simulink model "StepperMotorPullIn"  (R2023b)
settings: Solver=ode23t  StartTime=0.0  StopTime=timeSimulation  FixedStep=0.001  MaxStep=1/(4*numMicroStep*f*4)  RelTol=1e-3  AbsTol=1e-3  EnableMultiTasking=on
PreLoadFcn:
  | % Parameterize the stepper motor;
  | StepperMotorPullInData;
values from neighbouring files (symbols this model uses):
  CF = sqrt(2)    [StepperMotorPullInData.m]
  driveRampRate = -1/log(1-(1-exp(-1))/voltageFactor)    [StepperMotorPullInData.m]
  f = stepRate/4    (= 75)    [StepperMotorPullInData.m]    (also in StepperMotorPullInUpdatePlot.m = stepRateVector(i)/4)
  fullStepSize = 1.8    [StepperMotorPullInData.m]    (also in StepperMotorPullin.mat)
  inductance = 4.6    [StepperMotorPullInData.m]
  LF = 1    [StepperMotorPullInData.m]
  loadDamping = 0    [StepperMotorPullInData.m]
  loadTorque = 125    [StepperMotorPullInData.m]    (also in StepperMotorPullInUpdatePlot.m = (loadTorqueHigh+loadTorqueLow)/2)
  numMicroStep = 24    [StepperMotorPullInData.m]
  ratedCurrent = 1.2    [StepperMotorPullInData.m]
  resistance = 2.2    [StepperMotorPullInData.m]
  rotorDamping = 0.1e-3    (= 0.0001)    [StepperMotorPullInData.m]
  rotorInertia = 37e-7    (= 3.7e-06)    [StepperMotorPullInData.m]
  tolerance = 2    [StepperMotorPullInData.m]
libraries: fl_lib x16, nesl_utility x7, simulink x1, ee_lib x1
CloseFcn:
  | try,close(figHandleMotorStepper),end
  | clear figHandleMotorStepper
  | 
  | try,close(figHandlePlotMotorStepper),end
  | clear figHandlePlotMotorStepper;
  | 
  | clear simlog_StepperMotorPullin;
  | 
  | clear modelFileName ratedCurrent ratedVoltage resistance;
  | clear inductance fullStepSize holdingTorque detentTorque;
  | clear rotorInertia kTVal rotorDamping initialSpeed;
  | clear initialAngle numMicroStep driveVoltage voltageFactor;
  | clear driveRampRate CF loadDamping loadInertia;
  | clear LF numRotation tolerance torqueTolerance stepRateVector f;
  | clear plotXAxis stepRate loadTorque loadCycle numStep timeSimulation;
  | clear i nF torque stepRateVectorSimulated slipped;
  | clear loadTorqueLow loadTorqueHigh notFinished loadTorque;
  | clear torqueSingle stepRateVectorSingle figAxes;
  | clear strucAutoSaveOptions loadTorqueLowInitial loadTorqueHighInitial;
  | clear torqueDatasheet stepRateVectorDatasheet;
  | clear torqueSingle stepRateVectorSingle;
Description:
  | Stepper Motor Pull-in Characteristics
  | %
settings Model: Creator=The MathWorks, Inc.  LastModifiedBy=The MathWorks, Inc.
settings SolverCC: AlgebraicLoopSolver=TrustRegion
settings DataIOCC: MaxDataPoints=10000  SaveFormat=Array  SaveOutput=off  SignalLogging=off  DSMLogging=off  SaveTime=off  ReturnWorkspaceOutputs=off  SignalLoggingName=logsout_StepperMotor
settings OptimizationCC: ReuseModelBlockBuffer=off  ExpressionDepthLimit=2147483647  InitFltsAndDblsToZero=on  LifeSpan=inf
settings DebuggingCC: UnderspecifiedInitializationDetection=Classic  MergeDetectMultiDrivingBlocksExec=none  FcnCallInpInsideContextMsg=warning  UnconnectedInputMsg=warning  UnconnectedOutputMsg=warning  UnconnectedLineMsg=warning  StateNameClashWarn=warning  PregeneratedLibrarySubsystemCodeDiagnostic=none  SFUnexpectedBacktrackingDiag=warning  SFNoUnconditionalDefaultTransitionDiag=warning  SFExecutionAtInitializationDiag=none  ArithmeticOperatorsInVariantConditions=warning
settings HardwareCC: ProdBitPerPointer=32  ProdBitPerSizeT=32  ProdBitPerPtrDiffT=32  ProdLargestAtomicFloat=None  ProdIntDivRoundTo=Undefined  ProdEndianess=Unspecified  ProdWordSize=32  ProdHWDeviceType=32-bit Generic
settings ModelReferenceCC: EnableRefExpFcnMdlSchedulingChecks=on  PropagateSignalLabelsOutOfModel=off
settings SFSimCC: SimUseLocalCustomCode=off  CustomCodeUndefinedFunction=UseInterfaceOnly
settings RTWCC: RTWUseLocalCustomCode=off  DLArmComputeVersion=19.05
settings CodeAppCC: StateflowObjectComments=on
settings GRTTargetCC: TargetLangStandard=C89/C90 (ANSI)  CombineOutputUpdateFcns=off  GRTInterface=on
settings ConfigComp: CovScope=ReferencedModels  CovMetricSettings=dw  CovSaveCumulativeToWorkspaceVar=on  CovSaveSingleToWorkspaceVar=on  CovExternalEMLEnable=off  CovSFcnEnable=off
settings SimscapeCC: SimscapeLogType=all  SimscapeLogName=simlog_StepperMotorPullin  SimscapeLogLimitData=off

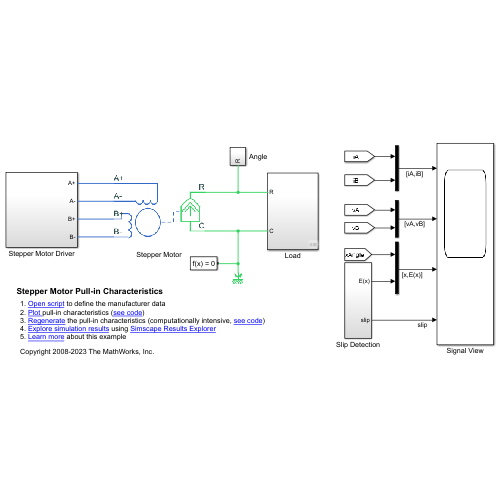
[thumbnail: Simulink's stored preview of the top-level diagram]
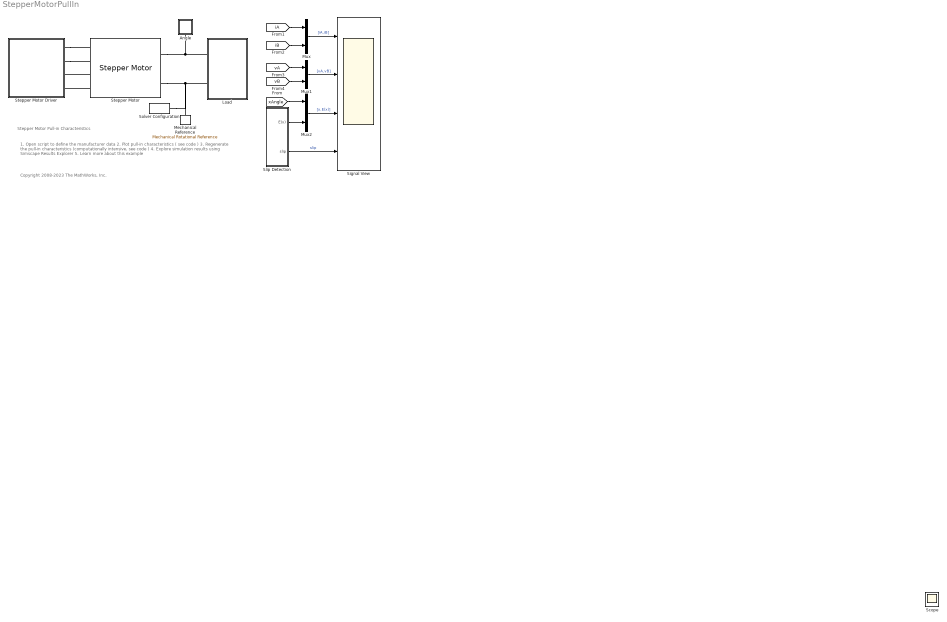
== system StepperMotorPullIn ==
  note: 1. Open script to define the manufacturer data
      | 2. Plot pull-in characteristics ( see code )
      | 3. Regenerate the pull-in characteristics (computationally intensive, see code )
      | 4. Explore simulation results using Simscape Results Explorer
      | 5. Learn more about this example
  note: Stepper Motor Pull-in Characteristics
  note: Copyright 2008-2023 The MathWorks, Inc.
  Angle : Subsystem
  Load : Subsystem
  Mechanical Reference : fl_lib/Mechanical/Rotational Elements/Mechanical Rotational Reference
  Mux : Mux  Inputs=2
  Mux1 : Mux  Inputs=2
  Mux2 : Mux  Inputs=2
  Signal View : Scope  NumInputPorts=4
  Slip Detection : Subsystem
  Solver Configuration : nesl_utility/Solver Configuration  PhysicalDomain=network_engine_domain  SubClassName=solver  LeftPortType=input  RightPortType=generic  Tones=[]  Harmonics=[]  SimulateNoise=off  Profile=off  UseLocalSampling=off  EnableSwitchedLinearOptims=on  FrequencyDomain=off  UseCCode=off  RelTol=0.001  AbsTol=1e-06  MinStep=1e-09  ToWorkspace=off  RevertToSquareIcSolve=off  NumHomotopyIterations=100  PhasorMode=off  PhasorModeNumHarmonics=1  ConsistencySolver=NEWTON_FTOL  IndexReductionMethod=DerivativeReplacement  DoDC=off  ResidualTolerance=1e-9  ConsistencyTolSource=GLOBAL  ConsistencyAbsTol=0.001  ConsistencyRelTol=0.001  ConsistencyTolFactor=0.001  UseLocalSolver=off  LocalSolverChoice=NE_BACKWARD_EULER_ADVANCER  ResolveIndetEquations=on  FunctionEvalNumThread=1  LocalSolverSampleTime=.001  DoFixedCost=off  MaxNonlinIter=3  MaxModeIter=2  ComputeImpulses=off  ImpulseIterations=2  LinearAlgebra=auto  LinearAlgebraNumThread=0  EquationFormulation=NE_TIME_EF  DelaysMemoryBudget=1024  AutomaticFiltering=off  FilteringTimeConstant=0.001  PartitionStorageMethod=AS_NEEDED  PartitionMemoryBudget=1024  PartitionMethod=FAST  MultibodyUseLocalSolver=off  MultibodyLocalSolverChoice=ODE1  MultibodyLocalSolverSampleTime=0.001
  Stepper Motor : ee_lib/Electromechanical/Reluctance & Stepper/Stepper Motor  step_or_av=1  Ra=resistance Ohm  La=inductance mH  Km=kTVal mN*m/A  Td=detentTorque mN*m  Rm=Inf Ohm  w_vec=[ 0 1000 3e+3 ] rpm  T_vec=[ 2 2 1 ] N*m  assert_if_slipping=0  J_total=1e-4 kg*m^2  max_step_rate=10 Hz  Step=fullStepSize deg  J=rotorInertia kg*m^2  B=rotorDamping N*m/(rad/s)  speed0=initialSpeed rpm  theta0=initialAngle deg  alpha=[.00393, .00393] 1/K  Tmeas=25 degC  Tmeas2=125 degC  T_vec2=[1.7, 1.7, .85] N*m  half_stepping=0  thermal_masses=[100, 100] J/K  initial_temperatures=[25, 25] degC  rotor_thermal_mass=50 J/K  rotor_initial_temperature=25 degC  Rm_percent_rotor=90
      settings: InternalSimscapePortConfiguration="{\"Bottom\":[],\"Left\":[{\"id\":\"pA\",\"label\":\"A+\",\"type\":\"foundation.electrical.electrical\"},{\"id\":\"nA\",\"label\":\"A-\",\"type\":\"foundation.electrical.electrical\"},{\"id\":\"pB\",\"label\":\"B+\",\"type\":\"foundation.electrical.electrical\"},{\"id\":\"nB\",\"label\":\"B-\",\"type\":\"foundation.electrical.electrical\"}],\"Right\":[{\"id\":\"R\",\"label\":\"R\",\"type\":\"foundation.mechanical.rotational.rotational\"},{\"id\":\"C\",\"label\":\"C\",\"type\":\"foundation.mechanical.rotational.rotational\"}],\"Top\":[]}"
  Stepper Motor Driver : Subsystem
  Scope : Scope
  wires:
  [vB] -> Mux1/2
  Mux1/1 -> Signal View/2  "[vA,vB]"
  [xAngle] -> Mux2/1
  Mux2/1 -> Signal View/3  "[x,E(x)]"
  Slip Detection/2(slip) -> Signal View/4  "slip"
  Mux/1 -> Signal View/1  "[iA,iB]"
  [iB] -> Mux/2
  [vA] -> Mux1/1
  [iA] -> Mux/1
  Slip Detection/1(E(x)) -> Mux2/2
  connections:
  Stepper Motor/RConn1 -- Load/LConn1 -- Angle/LConn1
  Stepper Motor/RConn2 -- Solver Configuration/RConn1 -- Mechanical Reference/LConn1 -- Load/LConn2
  Stepper Motor Driver/RConn1 -- Stepper Motor/LConn1
  Stepper Motor Driver/RConn2 -- Stepper Motor/LConn2
  Stepper Motor/LConn3 -- Stepper Motor Driver/RConn3
  Stepper Motor/LConn4 -- Stepper Motor Driver/RConn4

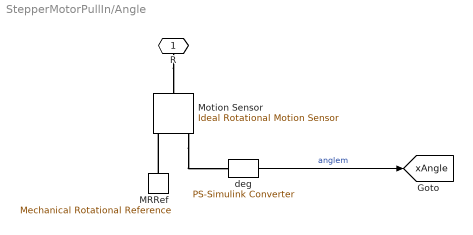
== system StepperMotorPullIn/Angle ==
  MRRef : fl_lib/Mechanical/Rotational Elements/Mechanical Rotational Reference
  Motion Sensor : fl_lib/Mechanical/Mechanical Sensors/Ideal Rotational Motion Sensor  reference=foundation.enum.MeasurementReference.difference  acceleration_port=false  velocity_port=true  position_port=true  wrap_angle=simscape.enum.onoff.off  offset=0 rad
  deg : nesl_utility/PS-Simulink Converter  PhysicalDomain=network_engine_domain  SubClassName=ps_output  LeftPortType=input  RightPortType=output  PseudoPeriodic=off  Frequencies=[]  VectorFormat=1-D array  Unit=deg  AffineConversion=off
  R : PMIOPort  Side=Left
  tag scope: xAngle=global
  wires:
  deg/1 -> [xAngle]  "anglem"
  connections:
  R/RConn1 -- Motion Sensor/LConn1
  Motion Sensor/RConn3 -- deg/LConn1
  MRRef/LConn1 -- Motion Sensor/RConn1

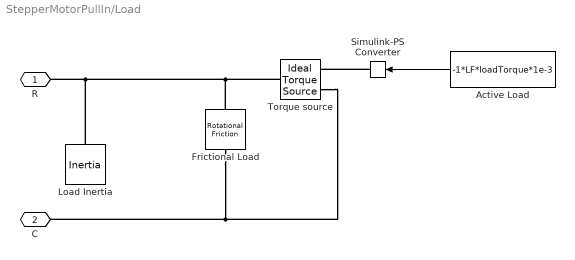
== system StepperMotorPullIn/Load ==
  Active Load : Constant  Value=-1*LF*loadTorque*1e-3
  Frictional Load : fl_lib/Mechanical/Rotational Elements/Rotational Friction  brkwy_trq=loadDamping+1.005*loadTorque*(1-LF)*1e-3+1e-7 N*m  brkwy_vel=0.02 rad/s  Col_trq=loadDamping+loadTorque*(1-LF)*1e-3+1e-8 N*m  visc_coef=(1e-9)*(1-LF)+0*0.001*(loadTorque+loadDamping)*(1-LF)*1e-3/(f*4*fullStepSize*pi/180) N*m/(rad/s)  w_specify=on  w_priority=None  w=initialSpeed rpm  w_nominal_specify=off  w_nominal_unit=rad/s  w_nominal_value=1  t_specify=off  t_priority=None  t=0 N*m  t_nominal_specify=off  t_nominal_unit=N*m  t_nominal_value=1
  Load Inertia : fl_lib/Mechanical/Rotational Elements/Inertia  inertia=loadInertia kg*m^2  num_ports=foundation.enum.numPorts2.one  w_specify=on  w_priority=High  w=initialSpeed rpm  w_nominal_specify=off  w_nominal_unit=rad/s  w_nominal_value=1  t_specify=off  t_priority=None  t=0 N*m  t_nominal_specify=off  t_nominal_unit=N*m  t_nominal_value=1
  Simulink-PS Converter : nesl_utility/Simulink-PS Converter  PhysicalDomain=network_engine_domain  SubClassName=ps_input  LeftPortType=input  RightPortType=output  PseudoPeriodic=off  Frequencies=[]  NoiseDistribution=none  NoiseParameters=[]  Unit=1  AffineConversion=off  FilteringAndDerivatives=provide  SimscapeFilterOrder=1  InputFilterTimeConstant=0.001  UdotUserProvided=0
  Torque source : fl_lib/Mechanical/Mechanical Sources/Ideal Torque Source
  R : PMIOPort  Side=Left
  C : PMIOPort  Port=2  Side=Left
  wires:
  Active Load/1 -> Simulink-PS Converter/1
  connections:
  Torque source/RConn2 -- C/RConn1 -- Frictional Load/RConn1
  Torque source/LConn1 -- Load Inertia/LConn1 -- R/RConn1 -- Frictional Load/LConn1
  Simulink-PS Converter/RConn1 -- Torque source/RConn1

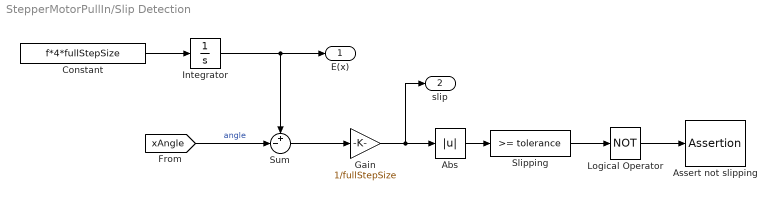
== system StepperMotorPullIn/Slip Detection ==
  Abs : Abs  ZeroCross=off  SaturateOnIntegerOverflow=off
  Assert not slipping : Assertion  AssertionFailFcn=disp('Stepper slipped')
  Constant : Constant  Value=f*4*fullStepSize
  Gain : Gain  Gain=1/fullStepSize
  Integrator : Integrator
  Logical Operator : Logic  Operator=NOT  AllPortsSameDT=off  OutDataTypeStr=boolean
  Slipping : simulink/Logic and Bit Operations/Compare To Constant  relop=>=  const=tolerance  OutDataTypeStr=boolean
  Sum : Sum  Inputs=+-|
  E(x) : Outport  VectorParamsAs1DForOutWhenUnconnected=off
  slip : Outport  Port=2  VectorParamsAs1DForOutWhenUnconnected=off
  wires:
  Constant/1 -> Integrator/1
  Integrator/1 -> E(x)/1, Sum/1
  [xAngle] -> Sum/2  "angle"
  Gain/1 -> slip/1, Abs/1
  Slipping/1 -> Logical Operator/1
  Logical Operator/1 -> Assert not slipping/1
  Sum/1 -> Gain/1
  Abs/1 -> Slipping/1

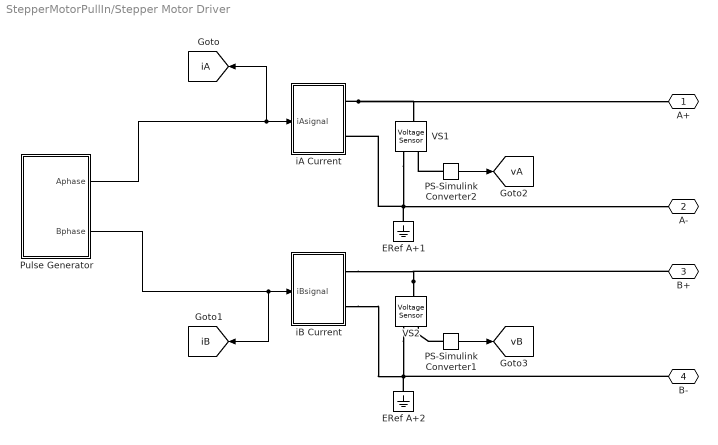
== system StepperMotorPullIn/Stepper Motor Driver ==
  ERef A+1 : fl_lib/Electrical/Electrical Elements/Electrical Reference
  ERef A+2 : fl_lib/Electrical/Electrical Elements/Electrical Reference
  PS-Simulink Converter1 : nesl_utility/PS-Simulink Converter  PhysicalDomain=network_engine_domain  SubClassName=ps_output  LeftPortType=input  RightPortType=output  PseudoPeriodic=off  Frequencies=[]  VectorFormat=1-D array  Unit=V  AffineConversion=off
  PS-Simulink Converter2 : nesl_utility/PS-Simulink Converter  PhysicalDomain=network_engine_domain  SubClassName=ps_output  LeftPortType=input  RightPortType=output  PseudoPeriodic=off  Frequencies=[]  VectorFormat=1-D array  Unit=V  AffineConversion=off
  Pulse Generator : Subsystem
  VS1 : fl_lib/Electrical/Electrical Sensors/Voltage Sensor
  VS2 : fl_lib/Electrical/Electrical Sensors/Voltage Sensor
  iA Current : Subsystem
  iB Current : Subsystem
  A+ : PMIOPort  Side=Right
  A- : PMIOPort  Port=2  Side=Right
  B+ : PMIOPort  Port=3  Side=Right
  B- : PMIOPort  Port=4  Side=Right
  tag scope: iA=global, iB=global, vA=global, vB=global
  wires:
  PS-Simulink Converter2/1 -> [vA]
  Pulse Generator/2(Bphase) -> [iB], iB Current/1(iBsignal)
  PS-Simulink Converter1/1 -> [vB]
  Pulse Generator/1(Aphase) -> [iA], iA Current/1(iAsignal)
  connections:
  VS2/RConn2 -- B-/RConn1 -- ERef A+2/LConn1 -- iB Current/RConn2
  PS-Simulink Converter1/LConn1 -- VS2/RConn1
  PS-Simulink Converter2/LConn1 -- VS1/RConn1
  VS2/LConn1 -- B+/RConn1 -- iB Current/RConn1
  iA Current/RConn1 -- A+/RConn1 -- VS1/LConn1
  VS1/RConn2 -- A-/RConn1 -- ERef A+1/LConn1 -- iA Current/RConn2

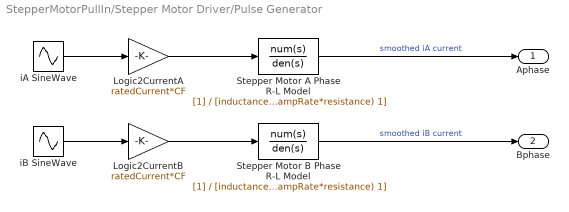
== system StepperMotorPullIn/Stepper Motor Driver/Pulse Generator ==
  Logic2CurrentA : Gain  Gain=ratedCurrent*CF
  Logic2CurrentB : Gain  Gain=ratedCurrent*CF
  Stepper Motor A Phase R-L Model : TransferFcn  Denominator=[inductance*1e-3/(driveRampRate*resistance) 1]
  Stepper Motor B Phase R-L Model : TransferFcn  Denominator=[inductance*1e-3/(driveRampRate*resistance) 1]
  iA SineWave : Sin  Frequency=2*pi*f  Phase=pi/2  SampleTime=1/(f*4*numMicroStep)
  iB SineWave : Sin  Frequency=2*pi*f  SampleTime=1/(f*4*numMicroStep)
  Aphase : Outport  VectorParamsAs1DForOutWhenUnconnected=off
  Bphase : Outport  Port=2  VectorParamsAs1DForOutWhenUnconnected=off
  wires:
  iA SineWave/1 -> Logic2CurrentA/1
  iB SineWave/1 -> Logic2CurrentB/1
  Stepper Motor A Phase R-L Model/1 -> Aphase/1  "smoothed iA current"
  Stepper Motor B Phase R-L Model/1 -> Bphase/1  "smoothed iB current"
  Logic2CurrentA/1 -> Stepper Motor A Phase R-L Model/1
  Logic2CurrentB/1 -> Stepper Motor B Phase R-L Model/1

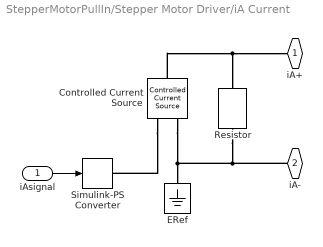
== system StepperMotorPullIn/Stepper Motor Driver/iA Current ==
  iAsignal : Inport
  Controlled Current Source : fl_lib/Electrical/Electrical Sources/Controlled Current Source
  ERef : fl_lib/Electrical/Electrical Elements/Electrical Reference
  Resistor : fl_lib/Electrical/Electrical Elements/Resistor  R=resistance*2000 Ohm  i_specify=off  i_priority=None  i=0 A  i_nominal_specify=off  i_nominal_unit=A  i_nominal_value=1  v_specify=off  v_priority=None  v=0 V  v_nominal_specify=off  v_nominal_unit=V  v_nominal_value=1
  Simulink-PS Converter : nesl_utility/Simulink-PS Converter  PhysicalDomain=network_engine_domain  SubClassName=ps_input  LeftPortType=input  RightPortType=output  PseudoPeriodic=off  Frequencies=[]  NoiseDistribution=none  NoiseParameters=[]  Unit=A  AffineConversion=off  FilteringAndDerivatives=zero  SimscapeFilterOrder=1  InputFilterTimeConstant=.001  UdotUserProvided=0
  iA+ : PMIOPort  Side=Right
  iA- : PMIOPort  Port=2  Side=Right
  wires:
  iAsignal/1 -> Simulink-PS Converter/1
  connections:
  Controlled Current Source/LConn1 -- iA+/RConn1 -- Resistor/LConn1
  iA-/RConn1 -- Resistor/RConn1 -- Controlled Current Source/RConn2 -- ERef/LConn1
  Controlled Current Source/RConn1 -- Simulink-PS Converter/RConn1

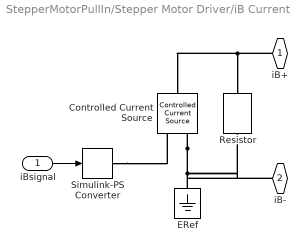
== system StepperMotorPullIn/Stepper Motor Driver/iB Current ==
  iBsignal : Inport
  Controlled Current Source : fl_lib/Electrical/Electrical Sources/Controlled Current Source
  ERef : fl_lib/Electrical/Electrical Elements/Electrical Reference
  Resistor : fl_lib/Electrical/Electrical Elements/Resistor  R=resistance*2000 Ohm  i_specify=off  i_priority=None  i=0 A  i_nominal_specify=off  i_nominal_unit=A  i_nominal_value=1  v_specify=off  v_priority=None  v=0 V  v_nominal_specify=off  v_nominal_unit=V  v_nominal_value=1
  Simulink-PS Converter : nesl_utility/Simulink-PS Converter  PhysicalDomain=network_engine_domain  SubClassName=ps_input  LeftPortType=input  RightPortType=output  PseudoPeriodic=off  Frequencies=[]  NoiseDistribution=none  NoiseParameters=[]  Unit=A  AffineConversion=off  FilteringAndDerivatives=zero  SimscapeFilterOrder=1  InputFilterTimeConstant=.001  UdotUserProvided=0
  iB+ : PMIOPort  Side=Right
  iB- : PMIOPort  Port=2  Side=Right
  wires:
  iBsignal/1 -> Simulink-PS Converter/1
  connections:
  Controlled Current Source/RConn2 -- iB-/RConn1 -- Resistor/RConn1 -- ERef/LConn1
  iB+/RConn1 -- Resistor/LConn1 -- Controlled Current Source/LConn1
  Simulink-PS Converter/RConn1 -- Controlled Current Source/RConn1
